simulink model "mpcACCsystem_2"  (R2022a)
settings: Solver=FixedStepAuto  StartTime=0.0  StopTime=T  RelTol=1e-3
values from neighbouring files (symbols this model uses):
  t_gap = 1.4    [PreRun.m]
  Ts = 0.1    [PreRun.m]
  v0_ego_1 = 20    [PreRun.m]
  v0_ego_2 = 20    [PreRun.m]
  v0_ego_3 = 20    [PreRun.m]
  v0_lead = 25    [PreRun.m]
  v_set = 30    [PreRun.m]
  x0_ego_1 = 38    [PreRun.m]
  x0_ego_2 = 0    [PreRun.m]
  x0_ego_3 = -38    [PreRun.m]
  x0_lead = 70    [PreRun.m]
libraries: mpcadaslib x3, eeStairGenerator x1
settings Model: Creator=The MathWorks, Inc.  LastModifiedBy=SAMEER TALWAR
settings SolverCC: AlgebraicLoopSolver=TrustRegion
settings DataIOCC: ReturnWorkspaceOutputs=off
settings DebuggingCC: UnconnectedInputMsg=warning  UnconnectedOutputMsg=warning  UnconnectedLineMsg=warning  SFMachineParentedDataDiag=warning  ArithmeticOperatorsInVariantConditions=warning
settings SFSimCC: SimUseLocalCustomCode=off  CustomCodeUndefinedFunction=UseInterfaceOnly
settings RTWCC: RTWUseLocalCustomCode=off
settings CodeAppCC: StateflowObjectComments=on

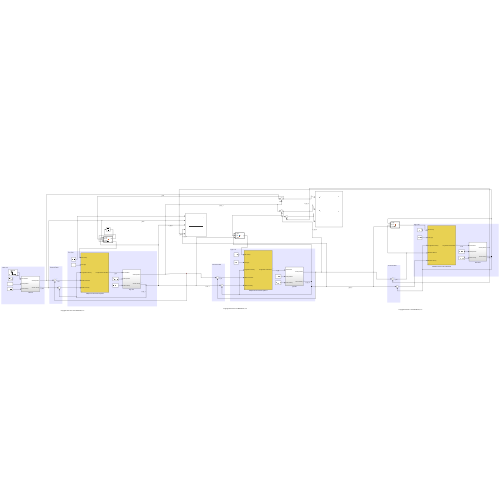
[thumbnail: Simulink's stored preview of the top-level diagram]
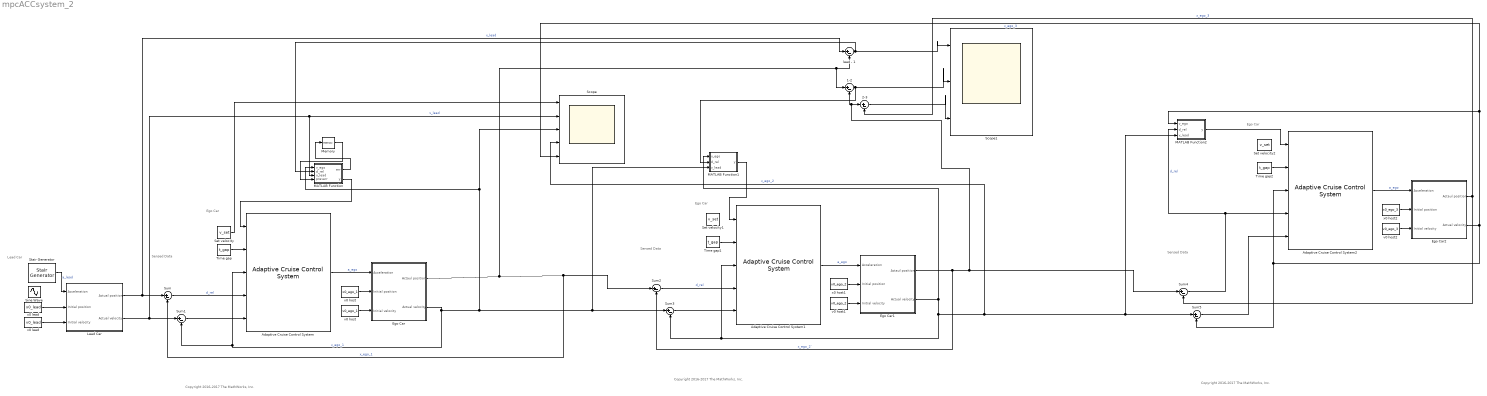
== system mpcACCsystem_2 ==
  note: Sensed Data
  note: Lead Car
  note: Ego Car
  note: Copyright 2016-2017 The MathWorks, Inc.
  note: Copyright 2016-2017 The MathWorks, Inc.
  note: Ego Car
  note: Sensed Data
  note: Sensed Data
  note: Copyright 2016-2017 The MathWorks, Inc.
  note: Ego Car
  1-2 : Sum  Inputs=|+-
  2-3 : Sum  Inputs=|+-
  Adaptive Cruise Control System : mpcadaslib/Adaptive Cruise Control System  EgoModel=tf(1,[0.5,1,0])  InitialEgoVelocity=20  DefaultSpacing=10  MaxVelocity=50  MinAcceleration=-3  amin_ext=off  MaxAcceleration=2  amax_ext=off  Ts=0.1  PredictionHorizon=30  ControllerBehavior=1.0  suboptimal=off  maxiter=10  datatypeopt=double  optmode=off  trackmode=off
  Adaptive Cruise Control System1 : mpcadaslib/Adaptive Cruise Control System  EgoModel=tf(1,[0.5,1,0])  InitialEgoVelocity=20  DefaultSpacing=10  MaxVelocity=50  MinAcceleration=-3  amin_ext=off  MaxAcceleration=2  amax_ext=off  Ts=0.1  PredictionHorizon=30  ControllerBehavior=1.0  suboptimal=off  maxiter=10  datatypeopt=double  optmode=off  trackmode=off
  Adaptive Cruise Control System2 : mpcadaslib/Adaptive Cruise Control System  EgoModel=tf(1,[0.5,1,0])  InitialEgoVelocity=20  DefaultSpacing=10  MaxVelocity=50  MinAcceleration=-3  amin_ext=off  MaxAcceleration=2  amax_ext=off  Ts=0.1  PredictionHorizon=30  ControllerBehavior=1.0  suboptimal=off  maxiter=10  datatypeopt=double  optmode=off  trackmode=off
  Ego Car : Subsystem
  Ego Car1 : Subsystem
  Ego Car2 : Subsystem
  Lead Car : Subsystem
  MATLAB Function : MATLAB Function  TreatAsAtomicUnit=on
  MATLAB Function1 : MATLAB Function  TreatAsAtomicUnit=on
  MATLAB Function2 : MATLAB Function  TreatAsAtomicUnit=on
  Memory : Memory
  Scope : Scope  NumInputPorts=5
  Scope1 : Scope  NumInputPorts=3
  Set velocity : Constant  Value=v_set  SampleTime=Ts
  Set velocity1 : Constant  Value=v_set  SampleTime=Ts
  Set velocity2 : Constant  Value=v_set  SampleTime=Ts
  Sine Wave : Sin  Amplitude=0.6  Frequency=0.2  SampleTime=Ts
  Stair Generator : eeStairGenerator/Stair Generator  LabelModeActiveChoice=Discrete  TimeInput=[55 60 70]  AmplitudeInput=[5 -2.5 0 ]  SampleTime=Ts  RepeatPattern=off  OutDataTypeStr=double
      settings: SourceProductBaseCode=PS
  Sum{,1..5} (6 alike) : Sum  Inputs=|+-
  Time gap : Constant  Value=t_gap  SampleTime=Ts
  Time gap1 : Constant  Value=t_gap  SampleTime=Ts
  Time gap2 : Constant  Value=t_gap  SampleTime=Ts
  lead - 1 : Sum  Inputs=|+-
  v0 host : Constant  Value=v0_ego_1  SampleTime=Ts
  v0 host1 : Constant  Value=v0_ego_2  SampleTime=Ts
  v0 host2 : Constant  Value=v0_ego_3  SampleTime=Ts
  v0 lead : Constant  Value=v0_lead  SampleTime=Ts
  x0 host : Constant  Value=x0_ego_1  SampleTime=Ts
  x0 host1 : Constant  Value=x0_ego_2  SampleTime=Ts
  x0 host2 : Constant  Value=x0_ego_3  SampleTime=Ts
  x0 lead : Constant  Value=x0_lead  SampleTime=Ts
  wires:
  x0 lead/1 -> Lead Car/2(Initial position)
  v0 lead/1 -> Lead Car/3(Initial velocity)
  x0 host/1 -> Ego Car/2(Initial position)
  Ego Car/2(Actual velocity) -> Adaptive Cruise Control System/3, Sum1/2, Scope/3, MATLAB Function/1(v_ego), MATLAB Function1/3(v_lead), Sum3/1  "v_ego_1"
  v0 host/1 -> Ego Car/3(Initial velocity)
  Adaptive Cruise Control System/1 -> Ego Car/1(Acceleration)  "a_ego"
  Lead Car/1(Actual position) -> lead - 1/1, Sum/1  "x_lead"
  Sum1/1 -> Adaptive Cruise Control System/5
  Time gap/1 -> Adaptive Cruise Control System/2
  Lead Car/2(Actual velocity) -> MATLAB Function/3(v_lead), Scope/2, Sum1/1  "v_lead"
  Sum/1 -> Adaptive Cruise Control System/4  "d_rel"
  Ego Car/1(Actaul position) -> lead - 1/2, 1-2/1, Sum2/1, Sum/2  "x_ego_1"
  v0 host1/1 -> Ego Car1/3(Initial velocity)
  x0 host1/1 -> Ego Car1/2(Initial position)
  Time gap1/1 -> Adaptive Cruise Control System1/2
  Sum2/1 -> Adaptive Cruise Control System1/4  "d_rel"
  Sum3/1 -> Adaptive Cruise Control System1/5
  Adaptive Cruise Control System1/1 -> Ego Car1/1(Acceleration)  "a_ego"
  Ego Car1/1(Actaul position) -> 1-2/2, 2-3/1, Sum4/1, Sum2/2  "x_ego_2'"
  v0 host2/1 -> Ego Car2/3(Initial velocity)
  x0 host2/1 -> Ego Car2/2(Initial position)
  Ego Car2/1(Actaul position) -> Sum4/2, 2-3/2  "x_ego_3"
  Ego Car2/2(Actual velocity) -> MATLAB Function2/1(v_ego), Scope/5, Adaptive Cruise Control System2/3, Sum5/2  "v_ego_3"
  Adaptive Cruise Control System2/1 -> Ego Car2/1(Acceleration)  "a_ego"
  Sum4/1 -> MATLAB Function2/2(d_rel), Adaptive Cruise Control System2/4  "d_rel"
  Time gap2/1 -> Adaptive Cruise Control System2/2
  Sum5/1 -> Adaptive Cruise Control System2/5
  Ego Car1/2(Actual velocity) -> MATLAB Function1/1(v_ego), Scope/4, MATLAB Function2/3(v_lead), Sum5/1, Adaptive Cruise Control System1/3, Sum3/2  "v_ego_2"
  Set velocity/1 -> Scope/1
  lead - 1/1 -> MATLAB Function/2(d_rel), Scope1/1
  1-2/1 -> MATLAB Function1/2(d_rel), Scope1/2
  2-3/1 -> Scope1/3
  MATLAB Function/2(y) -> Adaptive Cruise Control System/1
  MATLAB Function1/1(y) -> Adaptive Cruise Control System1/1
  MATLAB Function2/1(y) -> Adaptive Cruise Control System2/1
  Stair Generator/1 -> Lead Car/1(Acceleration)  "a_lead"
  MATLAB Function/1(err) -> Memory/1
  Memory/1 -> MATLAB Function/4(preverr)

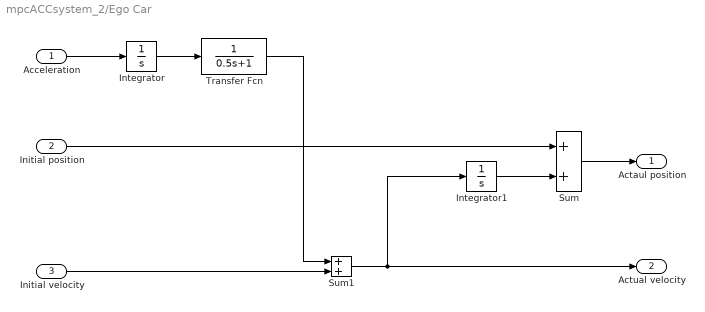
== system mpcACCsystem_2/Ego Car ==
  Acceleration : Inport
  Initial position : Inport  Port=2
  Initial velocity : Inport  Port=3
  Integrator : Integrator
  Integrator1 : Integrator
  Sum : Sum
  Sum1 : Sum
  Transfer Fcn : TransferFcn  Denominator=[0.5 1]
  Actaul position : Outport  VectorParamsAs1DForOutWhenUnconnected=off
  Actual velocity : Outport  Port=2  VectorParamsAs1DForOutWhenUnconnected=off
  wires:
  Sum1/1 -> Integrator1/1, Actual velocity/1
  Initial velocity/1 -> Sum1/2
  Sum/1 -> Actaul position/1
  Transfer Fcn/1 -> Sum1/1
  Integrator/1 -> Transfer Fcn/1
  Acceleration/1 -> Integrator/1
  Initial position/1 -> Sum/1
  Integrator1/1 -> Sum/2

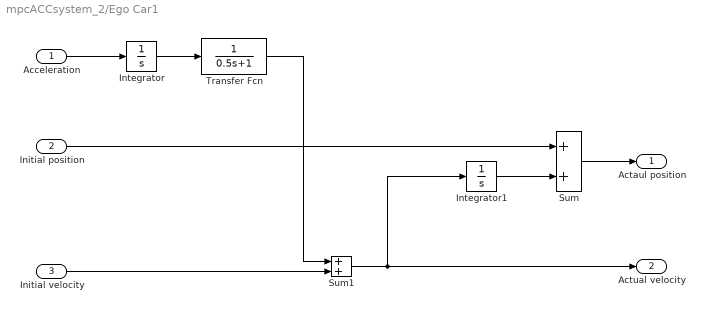
== system mpcACCsystem_2/Ego Car1 ==
  Acceleration : Inport
  Initial position : Inport  Port=2
  Initial velocity : Inport  Port=3
  Integrator : Integrator
  Integrator1 : Integrator
  Sum : Sum
  Sum1 : Sum
  Transfer Fcn : TransferFcn  Denominator=[0.5 1]
  Actaul position : Outport  VectorParamsAs1DForOutWhenUnconnected=off
  Actual velocity : Outport  Port=2  VectorParamsAs1DForOutWhenUnconnected=off
  wires:
  Sum1/1 -> Integrator1/1, Actual velocity/1
  Initial velocity/1 -> Sum1/2
  Sum/1 -> Actaul position/1
  Transfer Fcn/1 -> Sum1/1
  Integrator/1 -> Transfer Fcn/1
  Acceleration/1 -> Integrator/1
  Initial position/1 -> Sum/1
  Integrator1/1 -> Sum/2

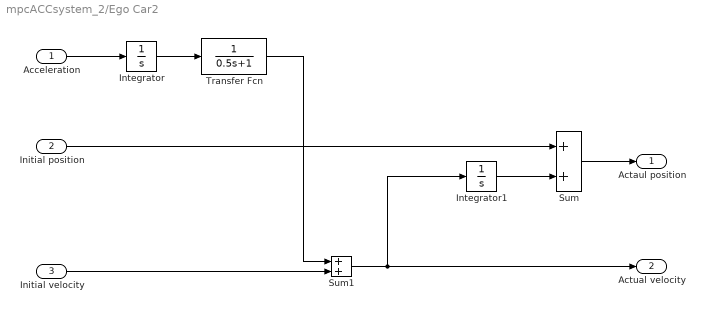
== system mpcACCsystem_2/Ego Car2 ==
  Acceleration : Inport
  Initial position : Inport  Port=2
  Initial velocity : Inport  Port=3
  Integrator : Integrator
  Integrator1 : Integrator
  Sum : Sum
  Sum1 : Sum
  Transfer Fcn : TransferFcn  Denominator=[0.5 1]
  Actaul position : Outport  VectorParamsAs1DForOutWhenUnconnected=off
  Actual velocity : Outport  Port=2  VectorParamsAs1DForOutWhenUnconnected=off
  wires:
  Sum1/1 -> Integrator1/1, Actual velocity/1
  Initial velocity/1 -> Sum1/2
  Sum/1 -> Actaul position/1
  Transfer Fcn/1 -> Sum1/1
  Integrator/1 -> Transfer Fcn/1
  Acceleration/1 -> Integrator/1
  Initial position/1 -> Sum/1
  Integrator1/1 -> Sum/2

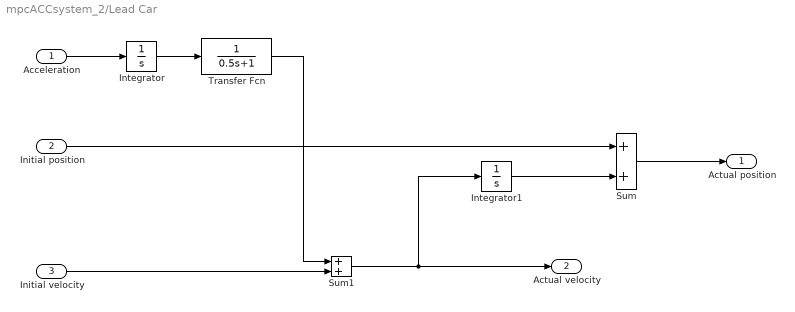
== system mpcACCsystem_2/Lead Car ==
  Acceleration : Inport
  Initial position : Inport  Port=2
  Initial velocity : Inport  Port=3
  Integrator : Integrator
  Integrator1 : Integrator
  Sum : Sum
  Sum1 : Sum
  Transfer Fcn : TransferFcn  Denominator=[0.5 1]
  Actual position : Outport  VectorParamsAs1DForOutWhenUnconnected=off
  Actual velocity : Outport  Port=2  VectorParamsAs1DForOutWhenUnconnected=off
  wires:
  Transfer Fcn/1 -> Sum1/1
  Initial velocity/1 -> Sum1/2
  Sum/1 -> Actual position/1
  Integrator/1 -> Transfer Fcn/1
  Sum1/1 -> Integrator1/1, Actual velocity/1
  Acceleration/1 -> Integrator/1
  Initial position/1 -> Sum/1
  Integrator1/1 -> Sum/2

== matlab function mpcACCsystem_2/MATLAB Function1 ==
  data: v_ego input; y output; d_rel input; v_lead input
function y = fcn(v_ego, d_rel, v_lead)
Kp = 1;
y = v_lead + Kp*(d_rel - (10 + (1.4*v_ego)));

== matlab function mpcACCsystem_2/MATLAB Function ==
  data: err output; v_ego input; y output; d_rel input; v_lead input; preverr input
function [err,y]= fcn(v_ego, d_rel, v_lead, preverr)
Kp = 5;
Kd = 0;
err = (d_rel - (10 + (1.4*v_ego)));
y = v_lead + Kp*err + Kd*(err-preverr);

== matlab function mpcACCsystem_2/MATLAB Function2 ==
  data: v_ego input; y output; d_rel input; v_lead input
function y = fcn(v_ego, d_rel, v_lead)
Kp = 1;
y = v_lead + Kp*(d_rel - (10 + (1.4*v_ego)));
